simulink model "serial_test_sim"  (R2019b)
settings: Solver=FixedStepAuto  StartTime=0.0625  StopTime=30  FixedStep=0.0625  RelTol=1e-3
undefined symbols (not defined in the file or in its folder): LF, serial
libraries: instrumentlib x3, sldrtlib x1
settings Model: Creator=bas  LastModifiedBy=bas

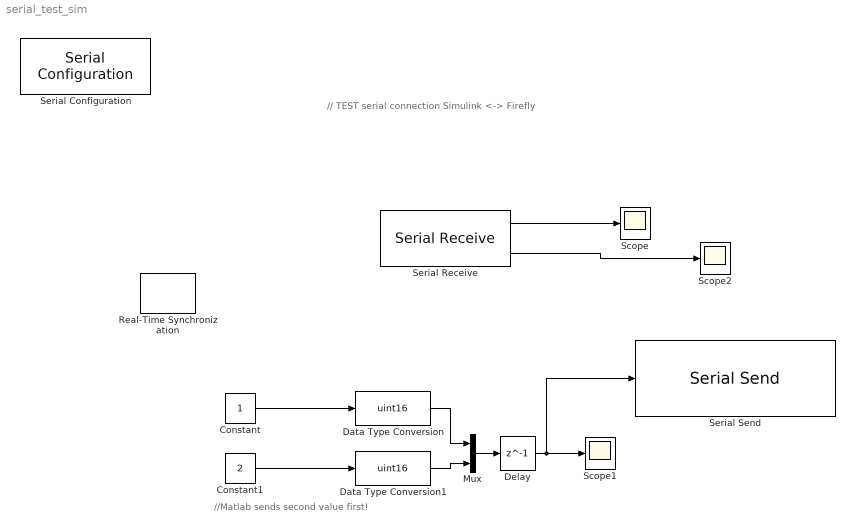
== system serial_test_sim ==
  note: //Matlab sends second value first!
  note: // TEST serial connection Simulink <-> Firefly
  Constant : Constant
  Constant1 : Constant  Value=2
  Data Type Conversion : DataTypeConversion  OutDataTypeStr=uint16
  Data Type Conversion1 : DataTypeConversion  OutDataTypeStr=uint16
  Delay : Delay  DelayLength=1
  Mux : Mux  Inputs=2
  Real-Time Synchronization : sldrtlib/Real-Time Synchronization  SampleTime=0.0625  MaxMissedTicks=10  ShowMissedTicks=off  YieldWhenWaiting=off
  Scope : Scope
  Scope1 : Scope
  Scope2 : Scope
  Serial Configuration : instrumentlib/Serial Configuration  Priority=-200000  ComPortMenu=/dev/cu.usbserial-141120  ComPort=/dev/cu.SLAB_USBtoUART  ObjConstructor=serial('/dev/cu.SLAB_USBtoUART');  BaudRate=460800  DataBits=8  Parity=none  StopBits=1  FlowControl=none  Timeout=10  ByteOrder=BigEndian
  Serial Receive : instrumentlib/Serial Receive  ComPortMenu=/dev/cu.SLAB_USBtoUART  ComPort=/dev/cu.SLAB_USBtoUART  ObjConstructor=serial('/dev/cu.SLAB_USBtoUART');  Terminator=LF ('\n')  DataSize="[2  1]"  DataType=uint16  EnableBlockingMode=off  ActionDataUnavailable=Output last received value  CustomValue=0  SampleTime=0.0625
  Serial Send : instrumentlib/Serial Send  ComPortMenu=/dev/cu.HookeVerse-SPPDev  ComPort=/dev/cu.SLAB_USBtoUART  ObjConstructor=serial('/dev/cu.SLAB_USBtoUART');  Header=#  Terminator=LF ('\n')  EnableBlockingMode=on
  wires:
  Serial Receive/1 -> Scope/1
  Delay/1 -> Serial Send/1, Scope1/1
  Serial Receive/2 -> Scope2/1
  Constant/1 -> Data Type Conversion/1
  Constant1/1 -> Data Type Conversion1/1
  Data Type Conversion/1 -> Mux/1
  Data Type Conversion1/1 -> Mux/2
  Mux/1 -> Delay/1
